simulink model "sst_llc_npc_inv"  (R2025b)
settings: Solver=ode23tb  StartTime=0.0  StopTime=simlength  FixedStep=tc  MaxStep=tc
values from neighbouring files (symbols this model uses):
  Adrso = eye(2) + Arso*ts_inv    [init_model.m]
  Aresd_max = eye(2) + Ares_max*ts_afe    [init_model.m]
  Aresd_min = eye(2) + Ares_min*ts_afe    [init_model.m]
  Aresd_nom = eye(2) + Ares_nom*ts_afe    [init_model.m]
  Bresd = Bres*ts_afe    [init_model.m]
  CFi_dc2 = 900e-6*4    (= 0.0036)    [init_model.m]
  Cresd = Cres    [init_model.m]
  Crso = [1 0]    [init_model.m]
  delta = 0.025    [init_model.m]
  fPWM_DAB = fPWM*4    (= 20000)    [init_model.m]
  freq = 50    [init_model.m]
  Iac_FS = I_phase_normalization_factor    [init_model.m]
  Idc_FS = max(Idab1_dc_nom,Idab2_dc_nom) * margin_factor    [init_model.m]
  iph_grid_pu_ref = 2.75    [init_model.m]
  ki_afe = 18    [init_model.m]
  ki_pll = 3140    [init_model.m]
  ki_rpi = 18    [init_model.m]
  kp_afe = 0.25    [init_model.m]
  kp_pll = 314    [init_model.m]
  kp_rpi = 0.25    [init_model.m]
  Ldrso = acker(Adrso',Crso',polesdrso)'    [init_model.m]
  LFu1_AFE = 0.33e-3    (= 0.00033)    [init_model.m]
  n_modules = 2    [init_model.m]
  RLFu1_AFE = 157*0.05*LFu1_AFE    (= 0.0025905)    [init_model.m]
  tc = ts_dab/1000*24    (= 1.2e-06)    [init_model.m]
  ts_afe = 1/fPWM_AFE    (= 0.0002)    [init_model.m]
  ts_inv = 1/fPWM_INV    (= 0.0002)    [init_model.m]
  Vac_FS = V_phase_normalization_factor    [init_model.m]
  Vdab2_dc_nom = 1500    [init_model.m]
  Vdc_FS = max(Vdab1_dc_nom,Vdab2_dc_nom) * margin_factor    [init_model.m]
undefined symbols (not defined in the file or in its folder): Ld2_trafo, omega_grid_nom, V_phase_normalization_factor
libraries: fl_lib x67, nesl_utility x39, full_bridge_mosfet_based_with_thermal_model x4, full_bridge_mosfet_based_with_thermal_model_zvs x4, pi_ctrl x4, discrete_time_low_pass_filter x4, full_bridge_three_level_npc_ideal_switch_based_model x3, single_phase_transformer x2, resonant_llc_modulator x2, full_bridge_ideal_switch x2, dclink_for_three_levels x2, full_bridge_three_level_npc_mosfet_based_model x2
(part 4 of 4)

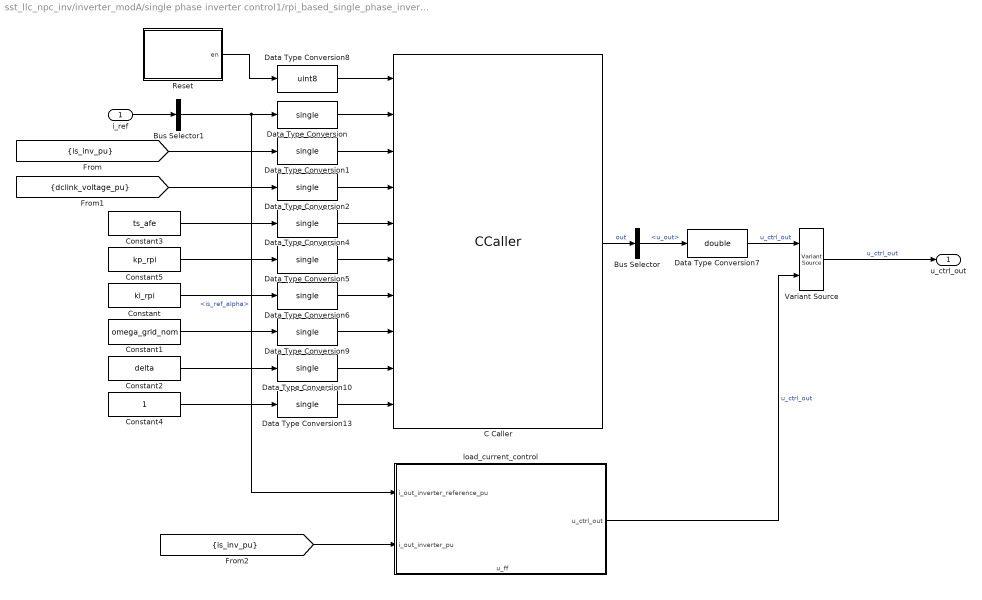
== system sst_llc_npc_inv/inverter_modA/single phase inverter control1/rpi_based_single_phase_inverter_ctrl/single_phase_current_control/rpi_current_controller ==
  i_ref : Inport
  Bus Selector : BusSelector  OutputSignals=u_out
  Bus Selector1 : BusSelector  OutputSignals=is_ref_alpha
  C Caller : CCaller  FunctionName=rpi_process_simulink  PortSpecificationStruct="%)30     .    V!(   8    (     @         %    \"     L    !     0         %  0 \"0    $    _    07)G3F%M90  4&]R=$YA;64 4V-O<&4     26YD97@     5'EP90      4VEZ90      27-';&]B86P   X    P    !@    @    $          4    (     0    ,    !         !   P!O=70 #@   #     &    \"     0         !0    @    !     P    $         $  # &]U=  .    .     8    (    !          %    \"     $    &     0         0   ...(+6126 chars)"
  Constant : Constant  Value=ki_rpi
  Constant1 : Constant  Value=omega_grid_nom
  Constant2 : Constant  Value=delta
  Constant3 : Constant  Value=ts_afe
  Constant4 : Constant
  Constant5 : Constant  Value=kp_rpi
  Data Type Conversion{,1..2,4..6,9..10,13} (9 alike) : DataTypeConversion  OutDataTypeStr=single  SaturateOnIntegerOverflow=off  RndMeth=Floor
  Data Type Conversion7 : DataTypeConversion  OutDataTypeStr=double  SaturateOnIntegerOverflow=off  RndMeth=Floor
  Data Type Conversion8 : DataTypeConversion  OutDataTypeStr=uint8  SaturateOnIntegerOverflow=off  RndMeth=Floor
  Reset : Subsystem
  Variant Source : VariantSource  VariantControls={rpi_ccaller == 1, rpi_ccaller == 0}
  load_current_control : Subsystem
      settings: PortSchema="{\"entries\":[{\"content\":{\"sides\":[{\"content\":{\"connectorIds\":[\"In1\",\"In2\"]},\"type\":\"ConnectorPlacement.EquallySpacedRectSide\",\"uuid\":\"b2775071-2eef-4aea-912c-3b123171bb94\"},{\"content\":{\"connectorIds\":[\"Out1\"],\"side\":\"RIGHT\"},\"type\":\"ConnectorPlacement.EquallySpacedRectSide\",\"uuid\":\"5b5540df-5797-4538-8091-e1ae4a6497c0\"},{\"content\":{\"side\":\"TOP\"},\"type\":\"ConnectorPlacement.EquallySpacedRectSide\",\"uuid\":\"e9f2386f-05bb-4d1a-869c-a946e0f509c1\"},{\"content\":{\"connectorIds\":[\"In3\"],\"side\":\"BOTTOM\"},\"type\":\"ConnectorPlacement.EquallySpacedRectSide\",\"uuid\":\"70f8ea50-374b-4030-9c25-af82787c8377\"}]},\"type\":\"ConnectorPlacement.EquallySpacedConnector\",\"uuid\":\"b6bc94ba-9f89-4502-b8f3-cff891faf17c\"}],\"packageUris\":[\"http://schema.mathworks.com/mf0/Connector/R2020b\"],\"version\":\"1.0\"}"
  u_ctrl_out : Outport
  wires:
  Constant4/1 -> Data Type Conversion13/1
  Constant2/1 -> Data Type Conversion10/1
  Constant1/1 -> Data Type Conversion9/1
  Constant/1 -> Data Type Conversion6/1
  Data Type Conversion8/1 -> C Caller/1
  Data Type Conversion/1 -> C Caller/2
  Data Type Conversion1/1 -> C Caller/3
  Data Type Conversion2/1 -> C Caller/4
  Data Type Conversion4/1 -> C Caller/5
  Data Type Conversion5/1 -> C Caller/6
  Data Type Conversion6/1 -> C Caller/7
  Data Type Conversion9/1 -> C Caller/8
  Data Type Conversion10/1 -> C Caller/9
  Data Type Conversion13/1 -> C Caller/10
  Constant3/1 -> Data Type Conversion4/1
  Constant5/1 -> Data Type Conversion5/1
  [dclink_voltage_pu] -> Data Type Conversion2/1
  [is_inv_pu] -> Data Type Conversion1/1
  i_ref/1 -> Bus Selector1/1
  Reset/1(en) -> Data Type Conversion8/1
  C Caller/1 -> Bus Selector/1  "out"
  Bus Selector/1 -> Data Type Conversion7/1  "<u_out>"
  Bus Selector1/1 -> load_current_control/1(i_out_inverter_reference_pu), Data Type Conversion/1  "<is_ref_alpha>"
  Data Type Conversion7/1 -> Variant Source/1  "u_ctrl_out"
  Variant Source/1 -> u_ctrl_out/1  "u_ctrl_out"
  load_current_control/1(u_ctrl_out) -> Variant Source/2  "u_ctrl_out"
  [is_inv_pu] -> load_current_control/2(i_out_inverter_pu)

== system sst_llc_npc_inv/inverter_modA/single phase inverter control1/rpi_based_single_phase_inverter_ctrl/single_phase_pll/double_integrator_observer ==
  theta : Inport
  Gain : Gain  Gain=Ldrso  Multiplication=Matrix(K*u)
  Gain1 : Gain  Gain=Adrso  Multiplication=Matrix(K*u)
  Gain2 : Gain  Gain=Crso  Multiplication=Matrix(K*u)
  Sum : Sum  Inputs=-+|
  Sum1 : Sum  Inputs=|++
  Unit Delay : UnitDelay  SampleTime=-1  HasFrameUpgradeWarning=on
  bounder1 : MATLAB Function  TreatAsAtomicUnit=on
  bounder2 : MATLAB Function  TreatAsAtomicUnit=on
  theta_hat : Outport
  wires:
  Gain/1 -> Sum1/1
  Gain2/1 -> bounder2/1(u)  "theta_hat"
  Gain1/1 -> Sum1/2
  Sum1/1 -> Unit Delay/1
  Sum/1 -> bounder1/1(u)  "e"
  Unit Delay/1 -> Gain1/1, Gain2/1
  theta/1 -> Sum/2  "theta"
  bounder1/1(y) -> Gain/1  "e_bounded"
  bounder2/1(y) -> theta_hat/1, Sum/1  "theta_hat_bounded"

== system sst_llc_npc_inv/inverter_modA/single phase inverter control1/rpi_based_single_phase_inverter_ctrl/single_phase_pll/pi-ctrl ==
  x : Inport
  xref : Inport  Port=2
  1/Ti : Gain  Gain=kp  SaturateOnIntegerOverflow=on  OutDataTypeStr=Inherit: Same as input  ParamDataTypeStr=Inherit: Same as input
  Saturation : Saturate  UpperLimit=sat_pos  LowerLimit=sat_neg
  Sum1 : Sum  Inputs=+++  SaturateOnIntegerOverflow=on
  Sum2 : Sum  Inputs=-+  SaturateOnIntegerOverflow=on
  Sum3 : Sum  Inputs=-+  SaturateOnIntegerOverflow=on
  Unit Delay4 : UnitDelay  SampleTime=-1  HasFrameUpgradeWarning=on
  kp : Gain  Gain=ki*ts  SaturateOnIntegerOverflow=on  OutDataTypeStr=Inherit: Same as input  ParamDataTypeStr=Inherit: Same as input
  u : Outport
  wires:
  Saturation/1 -> Sum3/2, u/1
  Unit Delay4/1 -> Sum1/3
  Sum1/1 -> Saturation/1
  Sum3/1 -> Unit Delay4/1
  1/Ti/1 -> Sum3/1, Sum1/1
  Sum2/1 -> 1/Ti/1, kp/1
  kp/1 -> Sum1/2
  x/1 -> Sum2/1
  xref/1 -> Sum2/2

== system sst_llc_npc_inv/inverter_modB/single phase inverter control1/rpi_based_single_phase_inverter_ctrl/single_phase_current_control/current_reference_generation ==
  mag_ref : Inport
  phase : Inport  Port=2
  Bus Creator : BusCreator  Inputs=2
  Product : Product
  Product1 : Product
  Sin : Trigonometry  Operator=cos
  Sin1 : Trigonometry
  is_ref : Outport
  idc_ref : Outport  Port=2
  wires:
  Sin/1 -> Product/2
  phase/1 -> Sin1/1, Sin/1
  mag_ref/1 -> idc_ref/1, Product1/1, Product/1
  Sin1/1 -> Product1/2
  Product/1 -> Bus Creator/1  "is_ref_alpha"
  Product1/1 -> Bus Creator/2  "is_ref_beta"
  Bus Creator/1 -> is_ref/1

== system sst_llc_npc_inv/inverter_modB/single phase inverter control1/rpi_based_single_phase_inverter_ctrl/single_phase_current_control/dqpi_current_controller ==
  i_ref : Inport
  alphabeta2dq : Subsystem
  dq2alphabeta : Subsystem
  dq_vector_pi : Subsystem
  i_alpha_beta : Scope  NumInputPorts=2
      settings: ActiveDisplayYMinimum=-6.1486700749010978  ActiveDisplayYMaximum=5.7726009866098824  DataLoggingVariableName=ScopeData2
  phase shift filter1 : phase_shift_filter/phase shift filter  f=omega_grid_nom/2/pi  ts=ts_afe
  u_out : Outport
  wires:
  dq2alphabeta/1(alpha) -> u_out/1
  [is_inv_pu] -> phase shift filter1/1, i_alpha_beta/1, alphabeta2dq/1(alpha)  "i_alpha"
  phase shift filter1/1 -> i_alpha_beta/2, alphabeta2dq/2(beta)  "i_beta"
  i_ref/1 -> dq_vector_pi/1(id_ref)  "id_ref"
  alphabeta2dq/1("d ") -> dq_vector_pi/2(id)  "id"
  alphabeta2dq/2("q ") -> dq_vector_pi/3(iq)  "iq"
  dq_vector_pi/1(ud_ctrl) -> dq2alphabeta/1(d)
  dq_vector_pi/2(uq_ctrl) -> dq2alphabeta/2(q)

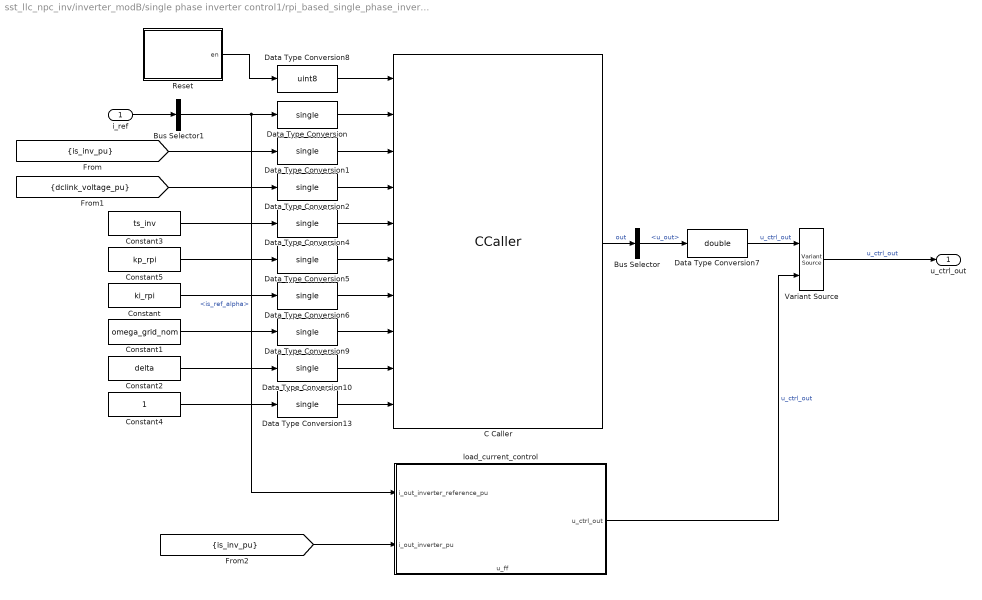
== system sst_llc_npc_inv/inverter_modB/single phase inverter control1/rpi_based_single_phase_inverter_ctrl/single_phase_current_control/rpi_current_controller ==
  i_ref : Inport
  Bus Selector : BusSelector  OutputSignals=u_out
  Bus Selector1 : BusSelector  OutputSignals=is_ref_alpha
  C Caller : CCaller  FunctionName=rpi_process_simulink  PortSpecificationStruct="%)30     .    V!(   8    (     @         %    \"     L    !     0         %  0 \"0    $    _    07)G3F%M90  4&]R=$YA;64 4V-O<&4     26YD97@     5'EP90      4VEZ90      27-';&]B86P   X    P    !@    @    $          4    (     0    ,    !         !   P!O=70 #@   #     &    \"     0         !0    @    !     P    $         $  # &]U=  .    .     8    (    !          %    \"     $    &     0         0   ...(+6126 chars)"
  Constant : Constant  Value=ki_rpi
  Constant1 : Constant  Value=omega_grid_nom
  Constant2 : Constant  Value=delta
  Constant3 : Constant  Value=ts_inv
  Constant4 : Constant
  Constant5 : Constant  Value=kp_rpi
  Data Type Conversion{,1..2,4..6,9..10,13} (9 alike) : DataTypeConversion  OutDataTypeStr=single  SaturateOnIntegerOverflow=off  RndMeth=Floor
  Data Type Conversion7 : DataTypeConversion  OutDataTypeStr=double  SaturateOnIntegerOverflow=off  RndMeth=Floor
  Data Type Conversion8 : DataTypeConversion  OutDataTypeStr=uint8  SaturateOnIntegerOverflow=off  RndMeth=Floor
  Reset : Subsystem
  Variant Source : VariantSource  VariantControls={rpi_ccaller == 1, rpi_ccaller == 0}
  load_current_control : Subsystem
      settings: PortSchema="{\"entries\":[{\"content\":{\"sides\":[{\"content\":{\"connectorIds\":[\"In1\",\"In2\"]},\"type\":\"ConnectorPlacement.EquallySpacedRectSide\",\"uuid\":\"b2775071-2eef-4aea-912c-3b123171bb94\"},{\"content\":{\"connectorIds\":[\"Out1\"],\"side\":\"RIGHT\"},\"type\":\"ConnectorPlacement.EquallySpacedRectSide\",\"uuid\":\"5b5540df-5797-4538-8091-e1ae4a6497c0\"},{\"content\":{\"side\":\"TOP\"},\"type\":\"ConnectorPlacement.EquallySpacedRectSide\",\"uuid\":\"e9f2386f-05bb-4d1a-869c-a946e0f509c1\"},{\"content\":{\"connectorIds\":[\"In3\"],\"side\":\"BOTTOM\"},\"type\":\"ConnectorPlacement.EquallySpacedRectSide\",\"uuid\":\"70f8ea50-374b-4030-9c25-af82787c8377\"}]},\"type\":\"ConnectorPlacement.EquallySpacedConnector\",\"uuid\":\"b6bc94ba-9f89-4502-b8f3-cff891faf17c\"}],\"packageUris\":[\"http://schema.mathworks.com/mf0/Connector/R2020b\"],\"version\":\"1.0\"}"
  u_ctrl_out : Outport
  wires:
  Constant4/1 -> Data Type Conversion13/1
  Constant2/1 -> Data Type Conversion10/1
  Constant1/1 -> Data Type Conversion9/1
  Constant/1 -> Data Type Conversion6/1
  Data Type Conversion8/1 -> C Caller/1
  Data Type Conversion/1 -> C Caller/2
  Data Type Conversion1/1 -> C Caller/3
  Data Type Conversion2/1 -> C Caller/4
  Data Type Conversion4/1 -> C Caller/5
  Data Type Conversion5/1 -> C Caller/6
  Data Type Conversion6/1 -> C Caller/7
  Data Type Conversion9/1 -> C Caller/8
  Data Type Conversion10/1 -> C Caller/9
  Data Type Conversion13/1 -> C Caller/10
  Constant3/1 -> Data Type Conversion4/1
  Constant5/1 -> Data Type Conversion5/1
  [dclink_voltage_pu] -> Data Type Conversion2/1
  [is_inv_pu] -> Data Type Conversion1/1
  i_ref/1 -> Bus Selector1/1
  Reset/1(en) -> Data Type Conversion8/1
  C Caller/1 -> Bus Selector/1  "out"
  Bus Selector/1 -> Data Type Conversion7/1  "<u_out>"
  Bus Selector1/1 -> load_current_control/1(i_out_inverter_reference_pu), Data Type Conversion/1  "<is_ref_alpha>"
  Data Type Conversion7/1 -> Variant Source/1  "u_ctrl_out"
  Variant Source/1 -> u_ctrl_out/1  "u_ctrl_out"
  load_current_control/1(u_ctrl_out) -> Variant Source/2  "u_ctrl_out"
  [is_inv_pu] -> load_current_control/2(i_out_inverter_pu)

== system sst_llc_npc_inv/inverter_modB/single phase inverter control1/rpi_based_single_phase_inverter_ctrl/single_phase_pll/double_integrator_observer ==
  theta : Inport
  Gain : Gain  Gain=Ldrso  Multiplication=Matrix(K*u)
  Gain1 : Gain  Gain=Adrso  Multiplication=Matrix(K*u)
  Gain2 : Gain  Gain=Crso  Multiplication=Matrix(K*u)
  Sum : Sum  Inputs=-+|
  Sum1 : Sum  Inputs=|++
  Unit Delay : UnitDelay  SampleTime=-1  HasFrameUpgradeWarning=on
  bounder1 : MATLAB Function  TreatAsAtomicUnit=on
  bounder2 : MATLAB Function  TreatAsAtomicUnit=on
  theta_hat : Outport
  wires:
  Gain/1 -> Sum1/1
  Gain2/1 -> bounder2/1(u)  "theta_hat"
  Gain1/1 -> Sum1/2
  Sum1/1 -> Unit Delay/1
  Sum/1 -> bounder1/1(u)  "e"
  Unit Delay/1 -> Gain1/1, Gain2/1
  theta/1 -> Sum/2  "theta"
  bounder1/1(y) -> Gain/1  "e_bounded"
  bounder2/1(y) -> theta_hat/1, Sum/1  "theta_hat_bounded"

== system sst_llc_npc_inv/inverter_modB/single phase inverter control1/rpi_based_single_phase_inverter_ctrl/single_phase_pll/pi-ctrl ==
  x : Inport
  xref : Inport  Port=2
  1/Ti : Gain  Gain=kp  SaturateOnIntegerOverflow=on  OutDataTypeStr=Inherit: Same as input  ParamDataTypeStr=Inherit: Same as input
  Saturation : Saturate  UpperLimit=sat_pos  LowerLimit=sat_neg
  Sum1 : Sum  Inputs=+++  SaturateOnIntegerOverflow=on
  Sum2 : Sum  Inputs=-+  SaturateOnIntegerOverflow=on
  Sum3 : Sum  Inputs=-+  SaturateOnIntegerOverflow=on
  Unit Delay4 : UnitDelay  SampleTime=-1  HasFrameUpgradeWarning=on
  kp : Gain  Gain=ki*ts  SaturateOnIntegerOverflow=on  OutDataTypeStr=Inherit: Same as input  ParamDataTypeStr=Inherit: Same as input
  u : Outport
  wires:
  Saturation/1 -> Sum3/2, u/1
  Unit Delay4/1 -> Sum1/3
  Sum1/1 -> Saturation/1
  Sum3/1 -> Unit Delay4/1
  1/Ti/1 -> Sum3/1, Sum1/1
  Sum2/1 -> 1/Ti/1, kp/1
  kp/1 -> Sum1/2
  x/1 -> Sum2/1
  xref/1 -> Sum2/2

== system sst_llc_npc_inv/inverter_modA/single phase inverter control1/rpi_based_single_phase_inverter_ctrl/single_phase_current_control/dqpi_current_controller/alphabeta2dq ==
  alpha : Inport
  beta : Inport  Port=2
  MATLAB Function : MATLAB Function  TreatAsAtomicUnit=on
  "d " : Outport  VectorParamsAs1DForOutWhenUnconnected=off
  "q " : Outport  Port=2  VectorParamsAs1DForOutWhenUnconnected=off
  wires:
  alpha/1 -> MATLAB Function/1(alpha)
  beta/1 -> MATLAB Function/2(beta)
  MATLAB Function/1(d) -> "d "/1
  MATLAB Function/2(q) -> "q "/1
  [phase] -> MATLAB Function/3(phase)

== system sst_llc_npc_inv/inverter_modA/single phase inverter control1/rpi_based_single_phase_inverter_ctrl/single_phase_current_control/dqpi_current_controller/dq2alphabeta ==
  d : Inport
  q : Inport  Port=2
  MATLAB Function : MATLAB Function  TreatAsAtomicUnit=on
  alpha : Outport  VectorParamsAs1DForOutWhenUnconnected=off
  wires:
  d/1 -> MATLAB Function/1(d)
  q/1 -> MATLAB Function/2(q)
  MATLAB Function/1(alpha) -> alpha/1
  [phase] -> MATLAB Function/3(phase)

== system sst_llc_npc_inv/inverter_modA/single phase inverter control1/rpi_based_single_phase_inverter_ctrl/single_phase_current_control/dqpi_current_controller/dq_vector_pi ==
  id_ref : Inport
  id : Inport  Port=2
  iq : Inport  Port=3
  Bus Creator : BusCreator  Inputs=3
  Bus Creator1 : BusCreator  Inputs=3
  Constant : Constant  Value=0
  dq_vector_pi : dq_vector_pi/dq_vector_pi  kp=kp_afe  ki=ki_afe  ts=ts_afe  lim_ctrl_out=1  CTRPIFF_CLIP_RELEASE=1e-3
  dq_vector_pi_tracking : Scope  NumInputPorts=2
      settings: ActiveDisplayYMinimum=-1.7699367830021773  ActiveDisplayYMaximum=2.6986467813918615  DataLoggingVariableName=ScopeData8
  ud_ctrl : Outport
  uq_ctrl : Outport  Port=2
  wires:
  id_ref/1 -> dq_vector_pi/1, Bus Creator/2  "id_ref"
  Constant/1 -> dq_vector_pi/3, Bus Creator1/1  "iq_ref"
  dq_vector_pi/1 -> ud_ctrl/1, Bus Creator/3  "ud_ctrl"
  iq/1 -> dq_vector_pi/4, Bus Creator1/2  "iq"
  id/1 -> dq_vector_pi/2, Bus Creator/1  "id"
  dq_vector_pi/2 -> uq_ctrl/1, Bus Creator1/3  "uq_ctrl"
  Bus Creator/1 -> dq_vector_pi_tracking/1
  Bus Creator1/1 -> dq_vector_pi_tracking/2
  [dclink_voltage_pu] -> dq_vector_pi/5

== system sst_llc_npc_inv/inverter_modA/single phase inverter control1/rpi_based_single_phase_inverter_ctrl/single_phase_current_control/rpi_current_controller/Reset ==
  Step : Step  Time=0.05  Before=1  After=0
  en : Outport
  wires:
  Step/1 -> en/1

== system sst_llc_npc_inv/inverter_modA/single phase inverter control1/rpi_based_single_phase_inverter_ctrl/single_phase_current_control/rpi_current_controller/load_current_control ==
  i_out_inverter_reference_pu : Inport
  i_out_inverter_pu : Inport  Port=2
  u_ff : Inport  Port=3
  Add : Sum  Inputs=+++
  Add1 : Sum  Inputs=+++
  Gain : Gain  Gain=kp_afe
  Gain1 : Gain  Gain=ki_afe
  Sum : Sum  Inputs=|+-
  res_max : Subsystem
  res_min : Subsystem
  res_nom : Subsystem
  u_ctrl_out : Outport
  wires:
  i_out_inverter_reference_pu/1 -> Sum/1  "is_ref"
  i_out_inverter_pu/1 -> Sum/2  "is"
  Add/1 -> u_ctrl_out/1  "u_ctrl_out"
  Sum/1 -> Gain1/1, Gain/1
  Gain/1 -> Add/1
  Gain1/1 -> res_max/1(u(k)), res_min/1(u(k)), res_nom/1(u(k))
  res_nom/1(y(k)) -> Add1/1
  res_min/1(y(k)) -> Add1/2
  res_max/1(y(k)) -> Add1/3
  Add1/1 -> Add/2
  u_ff/1 -> Add/3

== system sst_llc_npc_inv/inverter_modB/single phase inverter control1/rpi_based_single_phase_inverter_ctrl/single_phase_current_control/dqpi_current_controller/alphabeta2dq ==
  alpha : Inport
  beta : Inport  Port=2
  MATLAB Function : MATLAB Function  TreatAsAtomicUnit=on
  "d " : Outport  VectorParamsAs1DForOutWhenUnconnected=off
  "q " : Outport  Port=2  VectorParamsAs1DForOutWhenUnconnected=off
  wires:
  alpha/1 -> MATLAB Function/1(alpha)
  beta/1 -> MATLAB Function/2(beta)
  MATLAB Function/1(d) -> "d "/1
  MATLAB Function/2(q) -> "q "/1
  [phase] -> MATLAB Function/3(phase)

== system sst_llc_npc_inv/inverter_modB/single phase inverter control1/rpi_based_single_phase_inverter_ctrl/single_phase_current_control/dqpi_current_controller/dq2alphabeta ==
  d : Inport
  q : Inport  Port=2
  MATLAB Function : MATLAB Function  TreatAsAtomicUnit=on
  alpha : Outport  VectorParamsAs1DForOutWhenUnconnected=off
  wires:
  d/1 -> MATLAB Function/1(d)
  q/1 -> MATLAB Function/2(q)
  MATLAB Function/1(alpha) -> alpha/1
  [phase] -> MATLAB Function/3(phase)

== system sst_llc_npc_inv/inverter_modB/single phase inverter control1/rpi_based_single_phase_inverter_ctrl/single_phase_current_control/dqpi_current_controller/dq_vector_pi ==
  id_ref : Inport
  id : Inport  Port=2
  iq : Inport  Port=3
  Bus Creator : BusCreator  Inputs=3
  Bus Creator1 : BusCreator  Inputs=3
  Constant : Constant  Value=0
  dq_vector_pi : dq_vector_pi/dq_vector_pi  kp=kp_afe  ki=ki_afe  ts=ts_inv  lim_ctrl_out=1  CTRPIFF_CLIP_RELEASE=1e-3
  dq_vector_pi_tracking : Scope  NumInputPorts=2
      settings: ActiveDisplayYMinimum=-3.0654203812524772  ActiveDisplayYMaximum=3.1263632436156286  DataLoggingVariableName=ScopeData8
  ud_ctrl : Outport
  uq_ctrl : Outport  Port=2
  wires:
  id_ref/1 -> dq_vector_pi/1, Bus Creator/2  "id_ref"
  Constant/1 -> dq_vector_pi/3, Bus Creator1/1  "iq_ref"
  dq_vector_pi/1 -> ud_ctrl/1, Bus Creator/3  "ud_ctrl"
  iq/1 -> dq_vector_pi/4, Bus Creator1/2  "iq"
  id/1 -> dq_vector_pi/2, Bus Creator/1  "id"
  dq_vector_pi/2 -> uq_ctrl/1, Bus Creator1/3  "uq_ctrl"
  Bus Creator/1 -> dq_vector_pi_tracking/1
  Bus Creator1/1 -> dq_vector_pi_tracking/2
  [dclink_voltage_pu] -> dq_vector_pi/5

== system sst_llc_npc_inv/inverter_modB/single phase inverter control1/rpi_based_single_phase_inverter_ctrl/single_phase_current_control/rpi_current_controller/Reset ==
  Step : Step  Time=0.05  Before=1  After=0
  en : Outport
  wires:
  Step/1 -> en/1

== system sst_llc_npc_inv/inverter_modB/single phase inverter control1/rpi_based_single_phase_inverter_ctrl/single_phase_current_control/rpi_current_controller/load_current_control ==
  i_out_inverter_reference_pu : Inport
  i_out_inverter_pu : Inport  Port=2
  u_ff : Inport  Port=3
  Add : Sum  Inputs=+++
  Add1 : Sum  Inputs=+++
  Gain : Gain  Gain=kp_afe
  Gain1 : Gain  Gain=ki_afe
  Sum : Sum  Inputs=|+-
  res_max : Subsystem
  res_min : Subsystem
  res_nom : Subsystem
  u_ctrl_out : Outport
  wires:
  i_out_inverter_reference_pu/1 -> Sum/1  "is_ref"
  i_out_inverter_pu/1 -> Sum/2  "is"
  Add/1 -> u_ctrl_out/1  "u_ctrl_out"
  Sum/1 -> Gain1/1, Gain/1
  Gain/1 -> Add/1
  Gain1/1 -> res_max/1(u(k)), res_min/1(u(k)), res_nom/1(u(k))
  res_nom/1(y(k)) -> Add1/1
  res_min/1(y(k)) -> Add1/2
  res_max/1(y(k)) -> Add1/3
  Add1/1 -> Add/2
  u_ff/1 -> Add/3

== system sst_llc_npc_inv/inverter_modA/single phase inverter control1/rpi_based_single_phase_inverter_ctrl/single_phase_current_control/rpi_current_controller/load_current_control/res_max ==
  u(k) : Inport
  Cresd : Gain  Gain=Cresd  Multiplication=Matrix(K*u)
  Gain2 : Gain  Gain=Bresd  Multiplication=Matrix(K*u)
  Gain3 : Gain  Gain=Aresd_max  Multiplication=Matrix(K*u)
  Sum2 : Sum  Inputs=|++  SaturateOnIntegerOverflow=on
  Unit Delay : UnitDelay  InitialCondition=[0 0]  SampleTime=-1  HasFrameUpgradeWarning=on
  y(k) : Outport
  wires:
  Sum2/1 -> Unit Delay/1  "x(k+1)"
  Gain3/1 -> Sum2/2
  Unit Delay/1 -> Gain3/1, Cresd/1  "x(k)"
  Gain2/1 -> Sum2/1
  Cresd/1 -> y(k)/1  "y(k)"
  u(k)/1 -> Gain2/1

== system sst_llc_npc_inv/inverter_modA/single phase inverter control1/rpi_based_single_phase_inverter_ctrl/single_phase_current_control/rpi_current_controller/load_current_control/res_min ==
  u(k) : Inport
  Cresd : Gain  Gain=Cresd  Multiplication=Matrix(K*u)
  Gain2 : Gain  Gain=Bresd  Multiplication=Matrix(K*u)
  Gain3 : Gain  Gain=Aresd_min  Multiplication=Matrix(K*u)
  Sum2 : Sum  Inputs=|++  SaturateOnIntegerOverflow=on
  Unit Delay : UnitDelay  InitialCondition=[0 0]  SampleTime=-1  HasFrameUpgradeWarning=on
  y(k) : Outport
  wires:
  u(k)/1 -> Gain2/1
  Cresd/1 -> y(k)/1  "y(k)"
  Gain2/1 -> Sum2/1
  Unit Delay/1 -> Cresd/1, Gain3/1  "x(k)"
  Gain3/1 -> Sum2/2
  Sum2/1 -> Unit Delay/1  "x(k+1)"

== system sst_llc_npc_inv/inverter_modA/single phase inverter control1/rpi_based_single_phase_inverter_ctrl/single_phase_current_control/rpi_current_controller/load_current_control/res_nom ==
  u(k) : Inport
  Cresd : Gain  Gain=Cresd  Multiplication=Matrix(K*u)
  Gain2 : Gain  Gain=Bresd  Multiplication=Matrix(K*u)
  Gain3 : Gain  Gain=Aresd_nom  Multiplication=Matrix(K*u)
  Sum2 : Sum  Inputs=|++  SaturateOnIntegerOverflow=on
  Unit Delay : UnitDelay  InitialCondition=[0 0]  SampleTime=-1  HasFrameUpgradeWarning=on
  y(k) : Outport
  wires:
  Sum2/1 -> Unit Delay/1  "x(k+1)"
  Gain3/1 -> Sum2/2
  Unit Delay/1 -> Gain3/1, Cresd/1  "x(k)"
  Gain2/1 -> Sum2/1
  Cresd/1 -> y(k)/1  "y(k)"
  u(k)/1 -> Gain2/1

== system sst_llc_npc_inv/inverter_modB/single phase inverter control1/rpi_based_single_phase_inverter_ctrl/single_phase_current_control/rpi_current_controller/load_current_control/res_max ==
  u(k) : Inport
  Cresd : Gain  Gain=Cresd  Multiplication=Matrix(K*u)
  Gain2 : Gain  Gain=Bresd  Multiplication=Matrix(K*u)
  Gain3 : Gain  Gain=Aresd_max  Multiplication=Matrix(K*u)
  Sum2 : Sum  Inputs=|++  SaturateOnIntegerOverflow=on
  Unit Delay : UnitDelay  InitialCondition=[0 0]  SampleTime=-1  HasFrameUpgradeWarning=on
  y(k) : Outport
  wires:
  Sum2/1 -> Unit Delay/1  "x(k+1)"
  Gain3/1 -> Sum2/2
  Unit Delay/1 -> Gain3/1, Cresd/1  "x(k)"
  Gain2/1 -> Sum2/1
  Cresd/1 -> y(k)/1  "y(k)"
  u(k)/1 -> Gain2/1

== system sst_llc_npc_inv/inverter_modB/single phase inverter control1/rpi_based_single_phase_inverter_ctrl/single_phase_current_control/rpi_current_controller/load_current_control/res_min ==
  u(k) : Inport
  Cresd : Gain  Gain=Cresd  Multiplication=Matrix(K*u)
  Gain2 : Gain  Gain=Bresd  Multiplication=Matrix(K*u)
  Gain3 : Gain  Gain=Aresd_min  Multiplication=Matrix(K*u)
  Sum2 : Sum  Inputs=|++  SaturateOnIntegerOverflow=on
  Unit Delay : UnitDelay  InitialCondition=[0 0]  SampleTime=-1  HasFrameUpgradeWarning=on
  y(k) : Outport
  wires:
  u(k)/1 -> Gain2/1
  Cresd/1 -> y(k)/1  "y(k)"
  Gain2/1 -> Sum2/1
  Unit Delay/1 -> Cresd/1, Gain3/1  "x(k)"
  Gain3/1 -> Sum2/2
  Sum2/1 -> Unit Delay/1  "x(k+1)"

== system sst_llc_npc_inv/inverter_modB/single phase inverter control1/rpi_based_single_phase_inverter_ctrl/single_phase_current_control/rpi_current_controller/load_current_control/res_nom ==
  u(k) : Inport
  Cresd : Gain  Gain=Cresd  Multiplication=Matrix(K*u)
  Gain2 : Gain  Gain=Bresd  Multiplication=Matrix(K*u)
  Gain3 : Gain  Gain=Aresd_nom  Multiplication=Matrix(K*u)
  Sum2 : Sum  Inputs=|++  SaturateOnIntegerOverflow=on
  Unit Delay : UnitDelay  InitialCondition=[0 0]  SampleTime=-1  HasFrameUpgradeWarning=on
  y(k) : Outport
  wires:
  Sum2/1 -> Unit Delay/1  "x(k+1)"
  Gain3/1 -> Sum2/2
  Unit Delay/1 -> Gain3/1, Cresd/1  "x(k)"
  Gain2/1 -> Sum2/1
  Cresd/1 -> y(k)/1  "y(k)"
  u(k)/1 -> Gain2/1

== matlab function sst_llc_npc_inv/inverter_modB/single phase inverter control1/rpi_based_single_phase_inverter_ctrl/single_phase_pll/double_integrator_observer/bounder1 ==
  data: u input; y output
function y = bounder(u)
    
    y = -pi + mod(u+3*pi,2*pi);
   
end

== matlab function sst_llc_npc_inv/inverter_modB/single phase inverter control1/rpi_based_single_phase_inverter_ctrl/single_phase_pll/double_integrator_observer/bounder2 ==
  data: u input; y output
function y = bounder(u)
    
    y = -pi + mod(u+3*pi,2*pi);
   
end

== matlab function sst_llc_npc_inv/inverter_modB/single phase inverter control1/rpi_based_single_phase_inverter_ctrl/single_phase_pll/xieta2alphabeta ==
  data: xi input; alpha output; eta input; gamma input; beta output
function [alpha,beta] = xieta2alphabeta(xi,eta,gamma)
    alpha  = xi*cos(gamma) - eta*sin(gamma);
    beta = xi*sin(gamma) + eta*cos(gamma);
end

== matlab function sst_llc_npc_inv/inverter_modA/single phase inverter control1/rpi_based_single_phase_inverter_ctrl/single_phase_pll/double_integrator_observer/bounder1 ==
  data: u input; y output
function y = bounder(u)
    
    y = -pi + mod(u+3*pi,2*pi);
   
end

== matlab function sst_llc_npc_inv/inverter_modA/single phase inverter control1/rpi_based_single_phase_inverter_ctrl/single_phase_pll/double_integrator_observer/bounder2 ==
  data: u input; y output
function y = bounder(u)
    
    y = -pi + mod(u+3*pi,2*pi);
   
end

== matlab function sst_llc_npc_inv/inverter_modA/single phase inverter control1/rpi_based_single_phase_inverter_ctrl/single_phase_pll/xieta2alphabeta ==
  data: xi input; alpha output; eta input; gamma input; beta output
function [alpha,beta] = xieta2alphabeta(xi,eta,gamma)
    alpha  = xi*cos(gamma) - eta*sin(gamma);
    beta = xi*sin(gamma) + eta*cos(gamma);
end

== matlab function sst_llc_npc_inv/line_source/phase_gen/bounder1 ==
  data: u input; y output
function y = bounder(u)
    
    y = -pi + mod(u+3*pi,2*pi);
end

== matlab function sst_llc_npc_inv/inverter_modB/single phase inverter control1/rpi_based_single_phase_inverter_ctrl/single_phase_current_control/dqpi_current_controller/alphabeta2dq/MATLAB Function ==
  data: alpha input; d output; beta input; phase input; q output
function [d, q] = alphabeta2dq(alpha, beta, phase)

d = alpha*cos(phase) + beta*sin(phase);
q = -alpha*sin(phase) + beta*cos(phase);

== matlab function sst_llc_npc_inv/inverter_modB/single phase inverter control1/rpi_based_single_phase_inverter_ctrl/single_phase_current_control/dqpi_current_controller/dq2alphabeta/MATLAB Function ==
  data: d input; alpha output; q input; phase input; beta output
function [alpha, beta] = dq2alphabeta(d, q, phase)

alpha = d*cos(phase) - q*sin(phase);
beta = d*sin(phase) + q*cos(phase);

== matlab function sst_llc_npc_inv/inverter_modB/single phase inverter control1/rpi_based_single_phase_inverter_ctrl/single_phase_pll/alphabeta2xieta ==
  data: alpha input; xi output; beta input; gamma input; eta output
function [xi,eta] = alphabeta2xieta(alpha,beta,gamma)
    xi  =  alpha*cos(gamma) + beta*sin(gamma);
    eta = -alpha*sin(gamma) + beta*cos(gamma);
end

== matlab function sst_llc_npc_inv/inverter_modA/single phase inverter control1/rpi_based_single_phase_inverter_ctrl/single_phase_pll/alphabeta2xieta ==
  data: alpha input; xi output; beta input; gamma input; eta output
function [xi,eta] = alphabeta2xieta(alpha,beta,gamma)
    xi  =  alpha*cos(gamma) + beta*sin(gamma);
    eta = -alpha*sin(gamma) + beta*cos(gamma);
end

== matlab function sst_llc_npc_inv/inverter_modA/single phase inverter control1/rpi_based_single_phase_inverter_ctrl/single_phase_current_control/dqpi_current_controller/alphabeta2dq/MATLAB Function ==
  data: alpha input; d output; beta input; phase input; q output
function [d, q] = alphabeta2dq(alpha, beta, phase)

d = alpha*cos(phase) + beta*sin(phase);
q = -alpha*sin(phase) + beta*cos(phase);

== matlab function sst_llc_npc_inv/inverter_modA/single phase inverter control1/rpi_based_single_phase_inverter_ctrl/single_phase_current_control/dqpi_current_controller/dq2alphabeta/MATLAB Function ==
  data: d input; alpha output; q input; phase input; beta output
function [alpha, beta] = dq2alphabeta(d, q, phase)

alpha = d*cos(phase) - q*sin(phase);
beta = d*sin(phase) + q*cos(phase);
